simulink model "SimulationKinematics"  (R2022b)
settings: Solver=VariableStepAuto  StartTime=0.0  StopTime=10.0  RelTol=1e-3
settings Model: Creator=vutie  LastModifiedBy=vutie

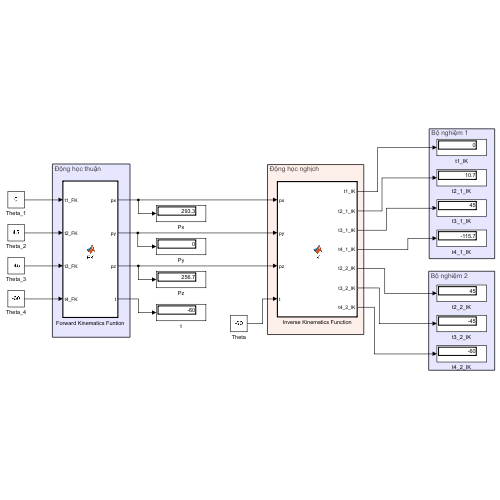
[thumbnail: Simulink's stored preview of the top-level diagram]
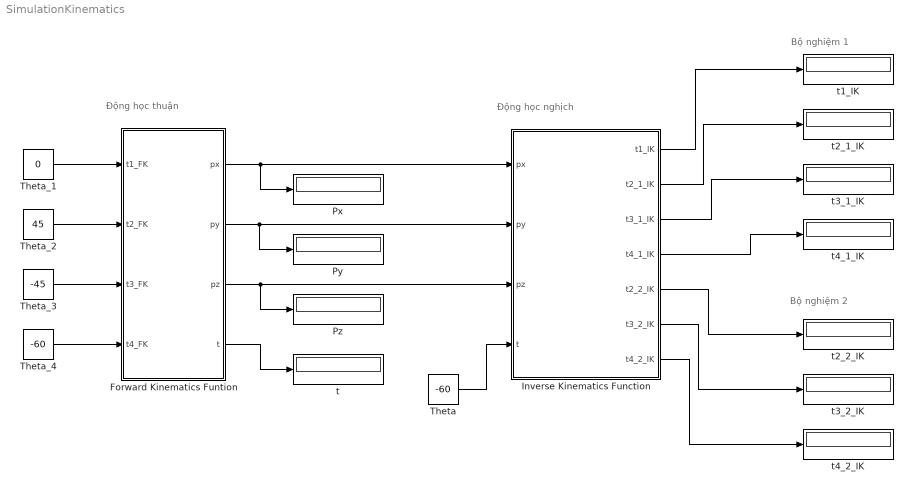
== system SimulationKinematics ==
  note: Động học thuận
  note: Động học nghịch
  note: Bộ nghiệm 1
  note: Bộ nghiệm 2
  Forward Kinematics Funtion : MATLAB Function  TreatAsAtomicUnit=on
  Inverse Kinematics Function : MATLAB Function  TreatAsAtomicUnit=on
  Px : Display
  Py : Display
  Pz : Display
  Theta : Constant  Value=-60
  Theta_1 : Constant  Value=0
  Theta_2 : Constant  Value=45
  Theta_3 : Constant  Value=-45
  Theta_4 : Constant  Value=-60
  t : Display
  t1_IK : Display
  "t2_1_IK " : Display
  t2_2_IK : Display
  t3_1_IK : Display
  t3_2_IK : Display
  t4_1_IK : Display
  t4_2_IK : Display
  wires:
  Theta_1/1 -> Forward Kinematics Funtion/1(t1_FK)
  Theta_3/1 -> Forward Kinematics Funtion/3(t3_FK)
  Theta_4/1 -> Forward Kinematics Funtion/4(t4_FK)
  Forward Kinematics Funtion/1(px) -> Px/1, Inverse Kinematics Function/1(px)
  Forward Kinematics Funtion/2(py) -> Py/1, Inverse Kinematics Function/2(py)
  Forward Kinematics Funtion/3(pz) -> Pz/1, Inverse Kinematics Function/3(pz)
  Forward Kinematics Funtion/4(t) -> t/1
  Inverse Kinematics Function/1(t1_IK) -> t1_IK/1
  Inverse Kinematics Function/2(t2_1_IK) -> "t2_1_IK "/1
  Inverse Kinematics Function/3(t3_1_IK) -> t3_1_IK/1
  Inverse Kinematics Function/4(t4_1_IK) -> t4_1_IK/1
  Inverse Kinematics Function/5(t2_2_IK) -> t2_2_IK/1
  Inverse Kinematics Function/6(t3_2_IK) -> t3_2_IK/1
  Inverse Kinematics Function/7(t4_2_IK) -> t4_2_IK/1
  Theta_2/1 -> Forward Kinematics Funtion/2(t2_FK)
  Theta/1 -> Inverse Kinematics Function/4(t)

== matlab function SimulationKinematics/Inverse Kinematics Function ==
  data: px input; t1_IK output; py input; pz input; t input; t2_1_IK output; t3_1_IK output; t4_1_IK output; t2_2_IK output; t3_2_IK output; t4_2_IK output
function [t1_IK,t2_1_IK,t3_1_IK,t4_1_IK,t2_2_IK,t3_2_IK,t4_2_IK] = IK(px,py,pz,t)
H = 62;
D1 = 176;
L1 = 91;
L2 = 122;
L3 = 77;
L4 = 78;

k = sqrt(px*px + py*py);
t1_IK = atan2d(py/k, px/k);
if(t1_IK < -180)
    t1_IK = t1_IK + 360;
end
if(t1_IK >= 180)
    t1_IK = t1_IK - 360;
end
E = px*cosd(t1_IK)+ py*sind(t1_IK) - L1 - L4*cosd(t);
F = pz-D1-H-L4*sind(t);
a = -2*L2*F;
b = -2*L2*E;
d = L3*L3 - E*E - F*F - L2*L2;
e = sqrt(a*a + b*b);
alpha = atan2d((-2*L2*F)/e, (-2*L2*E)/e);
atan2d(-sqrt(1-d*d/(e*e)), d/e)
t2_1_IK = atan2d(sqrt(1-d*d/(e*e)), d/e) + alpha;
if(t2_1_IK < -180)
    t2_1_IK = t2_1_IK + 360;
end
if(t2_1_IK >= 180)
    t2_1_IK = t2_1_IK - 360;
end
t2_2_IK = atan2d(-sqrt(1-d*d/(e*e)), d/e) + alpha;
if(t2_2_IK < -180)
    t2_2_IK = t2_2_IK + 360;
end
if(t2_2_IK >= 180)
    t2_2_IK = t2_2_IK - 360;
end
C23_1 = (px*cosd(t1_IK)+py*sind(t1_IK)-L1-L2*cosd(t2_1_IK)-L4*cosd(t))/L3;
S23_1 = (pz-D1-H-L2*sind(t2_1_IK)-L4*sind(t))/L3;
t3_1_IK = atan2d(S23_1, C23_1)-t2_1_IK;
if(t3_1_IK < -180)
    t3_1_IK = t3_1_IK + 360;
end
if(t3_1_IK >= 180)
    t3_1_IK = t2_1_IK - 360;
end
C23_2 = (px*cosd(t1_IK)+py*sind(t1_IK)-L1-L2*cosd(t2_2_IK)-L4*cosd(t))/L3;
S23_2 = (pz-D1-H-L2*sind(t2_2_IK)-L4*sind(t))/L3;
t3_2_IK = atan2d(S23_2, C23_2)-t2_2_IK;
if(t3_2_IK < -180)
    t3_2_IK = t3_2_IK + 360;
end
if(t3_2_IK >= 180)
    t3_2_IK = t3_2_IK - 360;
end
t4_1_IK = t - t2_1_IK - t3_1_IK;
t4_2_IK = t - t2_2_IK - t3_2_IK;

== matlab function SimulationKinematics/Forward Kinematics Funtion ==
  data: t1_FK input; px output; t2_FK input; t3_FK input; t4_FK input; py output; pz output; t output
function [px,py,pz,t] = FK(t1_FK,t2_FK,t3_FK,t4_FK)
H = 62;
D1 = 176;
L1 = 91;
L2 = 122;
L3 = 77;
L4 = 78;

t = t2_FK + t3_FK + t4_FK;
px = cosd(t1_FK)*(L1 + L2*cosd(t2_FK) + L3*cosd(t2_FK + t3_FK) + L4*cosd(t));
py = sind(t1_FK)*(L1 + L2*cosd(t2_FK) + L3*cosd(t2_FK + t3_FK) + L4*cosd(t));
pz = D1 + H + L3*sind(t2_FK + t3_FK) + L2*sind(t2_FK) + L4*sind(t);
